simulink model "GFo_LCL_Filter"  (R2015b)
settings: Solver=ode1  SolverMode=SingleTasking  StartTime=0.0  StopTime=15  FixedStep=Time_Step  MaxStep=1e-5  RelTol=1e-3
PreLoadFcn:
  | GFo_LCL_Filter_Init;
InitFcn:
  | GFo_LCL_Filter_Init;
undefined symbols (not defined in the file): L_1, L_2, R_1, R_2, Time_Step
libraries: powerlib x9, Source_Lib x1, GFo_Lib x1
settings Model: Creator=Frederic_Colas  LastModifiedBy=fcolas
settings DataIOCC: LimitDataPoints=off  SaveFormat=StructureWithTime
settings DebuggingCC: UnconnectedInputMsg=none  UnconnectedOutputMsg=none  UnconnectedLineMsg=none  AllowSymbolicDim=on  SFUnexpectedBacktrackingDiag=error  SFNoUnconditionalDefaultTransitionDiag=error
settings HardwareCC: ProdWordSize=32  ProdHWDeviceType=Specified
settings ModelReferenceCC: PropagateSignalLabelsOutOfModel=on
settings GRTTargetCC: TargetLangStandard=C99 (ISO)
settings ConfigComp: CovMetricSettings=dwe  CovSaveCumulativeToWorkspaceVar=off  CovSaveSingleToWorkspaceVar=off  CovModelRefEnable=Off  CovExternalEMLEnable=on
settings SimscapeCC: SimscapeNormalizeSystem=off

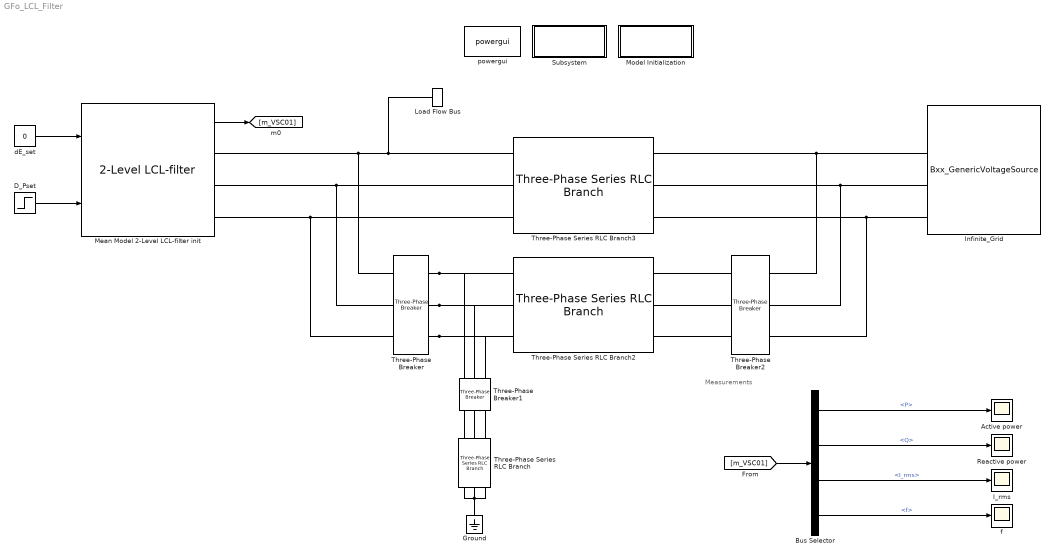
== system GFo_LCL_Filter ==
  note: Measurements
  Active power : Scope
  Bus Selector : BusSelector  OutputSignals=P,Q,VI.I_rms,f
  D_Pset : Step  Time=10.02  After=-0.8  SampleTime=0
  Ground : powerlib/Elements/Ground  LConnTagsString=a
  I_rms : Scope
  Infinite_Grid : Source_Lib/Bxx_GenericVoltageSource  SourceNature_str=INFINITE  fn=50  Sn=1e9  Un=GRD00_Un  LFpopup=Swing  P0=-778056837.7833  Q0=217569669.4637  V0_pu=1  U0=20000  Theta0_deg=0  H_s=5  DroopOnOff=on  R_percent=4  TN=1  TD=2
  Load Flow Bus : powerlib/Measurements/Load Flow Bus  LConnTagsString=a  Phases=single  Connectors=on one side  ID=BUS_1  Vbase=GRD00_Un  Vref=1  Vangle=0  VLF=0.99  VLFb=1  VLFc=1  angleLF=15.62  angleLFb=0  angleLFc=0
  Mean Model 2-Level LCL-filter init : GFo_Lib/2-Level LCL-filter  fn=50  Sn=1000e6  Pn=1000e6  Udcn=640e3  Time_Step=Time_Step  bridge_type=Average (no switches)  fpwm=4e3  Un1=320e3  Un2=400e3  Rt_pu=0.005  Lt_pu=0.15  Rm_pu=500  Lm_pu=500  Lf_pu=0.15  Rf_pu=0.005  Cf_pu=0.066  H_DC=40  Tr_PLL=10  Val_Freq_Support=on  Val_gamma=on  R_percent=4  Rv=0.09  W_TVR=60  I_thresh_pu=1.1  DX_DR=5  Kp_Rvi_pu=0.676  RLCL_D=0.7  f_damping=200  I_max_pu=1.2  Tr_I_max=100  Advanced=on  gainpopup=With Inertia  f_Inertia_Less=3  zeta_Inertia_Less=1  Param_Inertia=PI  H_GFo=3  zeta_GFo=0.7  LFpopup=PQ  P0=0.8  Q0=2.7756e-17  V0=0.99002  Theta0=15.6227
  Model Initialization : Subsystem  mask(Model Functions){InitFcnX=GFo_LCL_Filter_Init;, prel=on, posl=off, inif=on, strf=off}
      mask prompts: InitFcnX "Initialisation"; prel "Preload Function"; posl "PostLoad Function"; inif "InitFcn"; strf "StartFcn"
      mask init:
      | currentBlock = gcb;
      | root = bdroot(currentBlock);
      | 
      | if ~strcmp(get_param(root,'BlockDiagramType'),'library')
      |     if prel==1
      |         set_param(root, 'PreLoadFcn', InitFcnX);
      |     else
      |         set_param(root, 'PreLoadFcn', '');
      |     end
      |     if inif==1
      |         set_param(root, 'InitFcn', InitFcnX);
      |     else
      |         set_param(root, 'InitFcn', '');
      |     end
      |     if strf==1
      |         set_param(root, 'StartFcn', InitFcnX);
      |     else
      |         set_param(root, 'StartFcn', '');
      |     end
      |     if posl==1
      |         set_param(root, 'PostLoadFcn', InitFcnX);
      |     else
      |         set_param(root, 'PostLoadFcn', '');
      |     end
      | end
      | 
      | pos = get_param(currentBlock, 'Position');
      | width = pos(3) - pos(1); height = pos(4) - pos(2);
      | txt = [ upper(root) '\n' '- InitFcn. . . . . '  get_param(root, 'InitFcn') ];
      settings: CopyFcn=set_param(gcb,'LinkStatus','none')
      mask Display:
      | %text(5, height*0.5, txt, 'horizontalAlignment', 'left', 'verticalAlignment', 'middle') ;
      | color('blue'),disp('Initialization Function\nParameters')
  Reactive power : Scope
  Subsystem : Subsystem
      settings: OpenFcn=LoadFlow_VSC
      mask Display: color('blue'),disp('Update Loadflow')
  Three-Phase Series RLC Branch : powerlib/Elements/Three-Phase Series RLC Branch  LConnTagsString=A|B|C  RConnTagsString=A|B|C  BranchType=R  Resistance=1  Inductance=1e-3  Capacitance=1e-6  Measurements=None
  Three-Phase Series RLC Branch2 : powerlib/Elements/Three-Phase Series RLC Branch  LConnTagsString=A|B|C  RConnTagsString=A|B|C  BranchType=RL  Resistance=R_2  Inductance=L_2  Capacitance=1e-6  Measurements=None
  Three-Phase Series RLC Branch3 : powerlib/Elements/Three-Phase Series RLC Branch  LConnTagsString=A|B|C  RConnTagsString=A|B|C  BranchType=RL  Resistance=R_1  Inductance=L_1  Capacitance=1e-6  Measurements=None
  Three-Phase Breaker : powerlib/Elements/Three-Phase Breaker  InitialState=closed  SwitchA=on  SwitchB=on  SwitchC=on  SwitchTimes=[1.5 4]  External=off  BreakerResistance=0.01  SnubberResistance=1e6  SnubberCapacitance=inf  Measurements=None
  Three-Phase Breaker1 : powerlib/Elements/Three-Phase Breaker  InitialState=open  SwitchA=on  SwitchB=on  SwitchC=on  SwitchTimes=[10 10.2]  External=off  BreakerResistance=0.01  SnubberResistance=1e6  SnubberCapacitance=inf  Measurements=None
  Three-Phase Breaker2 : powerlib/Elements/Three-Phase Breaker  InitialState=closed  SwitchA=on  SwitchB=on  SwitchC=on  SwitchTimes=[1.5 4]  External=off  BreakerResistance=0.01  SnubberResistance=1e6  SnubberCapacitance=inf  Measurements=None
  dE_set : Constant  Value=0
  f : Scope
  powergui : powerlib/powergui  Priority=1  SimulationMode=Discrete  SampleTime=Time_Step  frequency=60  Iterations=50  frequencyindice=50  Pbase=1000000000  ErrMax=1e-6  UnitsV=kV  UnitsW=MW  buscounter=0  FunctionMessages=off  echomessages=off  EnableUseOfTLC=off  CurrentSourceSwitches=off  DisableSnubberDevices=off  DisableRonSwitches=off  DisableVfSwitches=off  DisplayEquations=off  AutomaticDiscreteSolvers=off  SolverType=Tustin/Backward Euler (TBE)  Interpol=off  ExternalGateDelay=off  methode=off  Ts=100  x0status=blocks  SPID=on  SwTol=0  HookPort=off  NonlinearTolerance=1e-4  nMaxIteration=100  ContinueOnMaxIteration=off  RestoreLinks=warning  ResistiveCurrentMeasurement=off  Frange=[0:2:500]  Ylog=off  Xlog=on  ShowGrid=off  save=off  variable=ZData  structure=0  ZoomFFT=off  StartTime=0.0  cycles=1  DisplayStyle=1  fundamental=60  FreqAxis=off  MaxFrequency=1000  frequencyindicesteady=1  RmsSteady=1  display=off
  wires:
  dE_set/1 -> Mean Model 2-Level LCL-filter init/1
  Mean Model 2-Level LCL-filter init/1 -> [m_VSC01]
  Bus Selector/1 -> Active power/1  "<P>"
  Bus Selector/2 -> Reactive power/1  "<Q>"
  [m_VSC01] -> Bus Selector/1
  Bus Selector/3 -> I_rms/1  "<I_rms>"
  D_Pset/1 -> Mean Model 2-Level LCL-filter init/2
  Bus Selector/4 -> f/1  "<f>"
  connections:
  Three-Phase Breaker/LConn1 -- Mean Model 2-Level LCL-filter init/RConn1 -- Load Flow Bus/LConn1 -- Three-Phase Series RLC Branch3/LConn1
  Three-Phase Breaker/LConn2 -- Mean Model 2-Level LCL-filter init/RConn2 -- Three-Phase Series RLC Branch3/LConn2
  Three-Phase Breaker/LConn3 -- Mean Model 2-Level LCL-filter init/RConn3 -- Three-Phase Series RLC Branch3/LConn3
  Three-Phase Breaker2/RConn2 -- Infinite_Grid/RConn2 -- Three-Phase Series RLC Branch3/RConn2
  Three-Phase Series RLC Branch/RConn2 -- Three-Phase Series RLC Branch/RConn3 -- Ground/LConn1 -- Three-Phase Series RLC Branch/RConn1
  Three-Phase Breaker/RConn3 -- Three-Phase Series RLC Branch2/LConn3 -- Three-Phase Breaker1/RConn3
  Three-Phase Breaker2/RConn1 -- Infinite_Grid/RConn1 -- Three-Phase Series RLC Branch3/RConn1
  Three-Phase Breaker2/RConn3 -- Infinite_Grid/RConn3 -- Three-Phase Series RLC Branch3/RConn3
  Three-Phase Breaker/RConn1 -- Three-Phase Series RLC Branch2/LConn1 -- Three-Phase Breaker1/RConn1
  Three-Phase Breaker/RConn2 -- Three-Phase Series RLC Branch2/LConn2 -- Three-Phase Breaker1/RConn2
  Three-Phase Series RLC Branch/LConn3 -- Three-Phase Breaker1/LConn3
  Three-Phase Breaker1/LConn2 -- Three-Phase Series RLC Branch/LConn2
  Three-Phase Series RLC Branch2/RConn3 -- Three-Phase Breaker2/LConn3
  Three-Phase Series RLC Branch2/RConn2 -- Three-Phase Breaker2/LConn2
  Three-Phase Series RLC Branch/LConn1 -- Three-Phase Breaker1/LConn1
  Three-Phase Series RLC Branch2/RConn1 -- Three-Phase Breaker2/LConn1

== system GFo_LCL_Filter/Model Initialization ==

== system GFo_LCL_Filter/Subsystem ==
